simulink model "Environmental_Model"  (R2016b)
settings: Solver=ode3  StartTime=0.0  StopTime=1500  RelTol=1e-3
InitFcn:
  | % Call parameters initialization function
  | run optiTruck_init_sim.m;
StopFcn:
  | %optiTruck_post_sim;
  | %optiTruck_plot_sim;
undefined symbols (not defined in the file or in its folder): kph_to_mps, Ts
settings Model: Creator=engin  LastModifiedBy=engin.ozatay
settings DataIOCC: SaveFormat=StructureWithTime  SaveOutput=off  SaveTime=off
settings OptimizationCC: BlockReduction=off  BufferReuse=off  LifeSpan=inf
settings DebuggingCC: AlgebraicLoopMsg=none  UnconnectedInputMsg=none  UnconnectedOutputMsg=none  UnconnectedLineMsg=none  SFExecutionAtInitializationDiag=none
settings HardwareCC: ProdBitPerSizeT=32  ProdBitPerPtrDiffT=32  ProdWordSize=32  ProdHWDeviceType=Specified

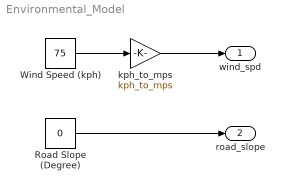
== system Environmental_Model ==
  Road Slope (Degree) : Constant  Value=0  SampleTime=Ts
  Wind Speed (kph) : Constant  Value=75  SampleTime=Ts
  kph_to_mps : Gain  Gain=kph_to_mps
  wind_spd : Outport  OutDataTypeStr=double  PortDimensions=1  SampleTime=[0.01,0]
  road_slope : Outport  Port=2  OutDataTypeStr=double  PortDimensions=1  SampleTime=[0.01,0]
  wires:
  kph_to_mps/1 -> wind_spd/1
  Wind Speed (kph)/1 -> kph_to_mps/1
  Road Slope (Degree)/1 -> road_slope/1
